simulink model "vaja3"  (R2020b)
settings: Solver=VariableStepAuto  StartTime=0.0  StopTime=142.3  RelTol=1e-3
values from neighbouring files (symbols this model uses):
  Ts = 0.1    [all_signals.m]    (also in cutting_signals.m; get_outputs.m; main_3.m; noise.m)
undefined symbols (not defined in the file or in its folder): U
libraries: PoKeysIOInterface x1
settings Model: Creator=64190198  LastModifiedBy=64190198

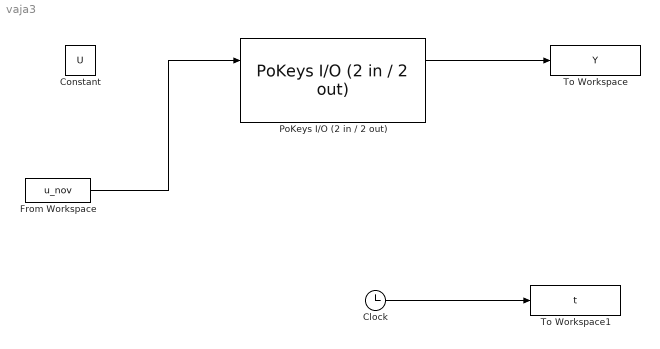
== system vaja3 ==
  Clock : Clock
  Constant : Constant  Value=U
  From Workspace : FromWorkspace  VariableName=u_nov
  PoKeys I/O (2 in / 2 out) : PoKeysIOInterface/PoKeys I//O (2 in // 2 out)  MaxPowerLimit=100.0  IOTs=Ts  IOSerial=500
      settings: SourceProductName=PoKeys I/O interface
  To Workspace : ToWorkspace  VariableName=Y  SampleTime=Ts
  To Workspace1 : ToWorkspace  VariableName=t  SampleTime=Ts
  wires:
  PoKeys I/O (2 in / 2 out)/1 -> To Workspace/1
  Clock/1 -> To Workspace1/1
  From Workspace/1 -> PoKeys I/O (2 in / 2 out)/1
